simulink model "Quad_Nonlinear_Pitch_Model"  (R2020a)
settings: Solver=ode4  StartTime=0.0  StopTime=5  FixedStep=0.01  RelTol=1e-3
InitFcn:
  | LQIR_Solver;
undefined symbols (not defined in the file or in its folder): B1, B5, Ba, K
settings Model: Creator=Ali  LastModifiedBy=Ali

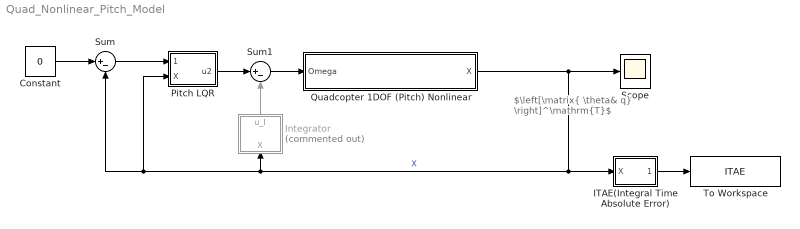
== system Quad_Nonlinear_Pitch_Model ==
  note: $\left[\matrix{ \theta& q} \right]^\mathrm{T}$
  Constant : Constant  Value=0
  ITAE(Integral Time Absolute Error) : Subsystem
  Integrator : Subsystem  Commented=on
  Pitch LQR : Subsystem
  Quadcopter 1DOF (Pitch) Nonlinear : Subsystem  TreatAsAtomicUnit=on
      mask Display: image('Seesaw.png'); % Use "Edit Image" on toolstrip to change.
  Scope : Scope
  Sum : Sum  Inputs=|+-
  Sum1 : Sum  Inputs=|+-
  To Workspace : ToWorkspace  VariableName=ITAE  SaveFormat=Timeseries  SampleTime=-1
  wires:
  Quadcopter 1DOF (Pitch) Nonlinear/1(X) -> Scope/1, Pitch LQR/2(X), Sum/2, Integrator/1(X), ITAE(Integral Time Absolute Error)/1(X)  "X"
  Constant/1 -> Sum/1
  Pitch LQR/1(u2) -> Sum1/1
  Sum1/1 -> Quadcopter 1DOF (Pitch) Nonlinear/1(Omega)
  Integrator/1(u_I) -> Sum1/2
  Sum/1 -> Pitch LQR/1(Error)
  ITAE(Integral Time Absolute Error)/1(ITAE) -> To Workspace/1

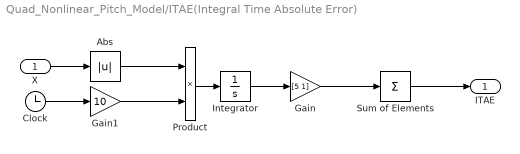
== system Quad_Nonlinear_Pitch_Model/ITAE(Integral Time Absolute Error) ==
  X : Inport
  Abs : Abs
  Clock : Clock
  Gain : Gain  Gain=[5 1]
  Gain1 : Gain  Gain=10
  Integrator : Integrator
  Product : Product
  Sum of Elements : Sum  Inputs=+
  ITAE : Outport
  wires:
  Product/1 -> Integrator/1
  Integrator/1 -> Gain/1
  Clock/1 -> Gain1/1
  Sum of Elements/1 -> ITAE/1
  Abs/1 -> Product/1
  X/1 -> Abs/1
  Gain/1 -> Sum of Elements/1
  Gain1/1 -> Product/2

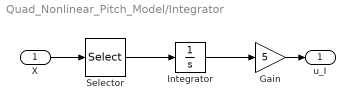
== system Quad_Nonlinear_Pitch_Model/Integrator ==
  X : Inport
  Gain : Gain  Gain=5
  Integrator : Integrator
  Selector : Selector  InputPortWidth=2  IndexOptions=Index vector (dialog)  Indices=[1]  OutputSizes=1
  u_I : Outport
  wires:
  Gain/1 -> u_I/1
  X/1 -> Selector/1
  Integrator/1 -> Gain/1
  Selector/1 -> Integrator/1

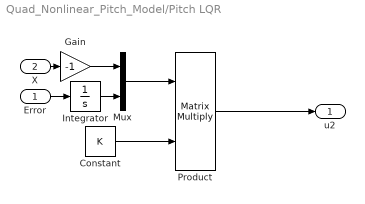
== system Quad_Nonlinear_Pitch_Model/Pitch LQR ==
  Error : Inport
  X : Inport  Port=2
  Constant : Constant  Value=K
  Gain : Gain  Gain=-1
  Integrator : Integrator
  Mux : Mux  Inputs=2
  Product : Product  Multiplication=Matrix(*)
  u2 : Outport
  wires:
  Product/1 -> u2/1
  X/1 -> Gain/1
  Error/1 -> Integrator/1
  Mux/1 -> Product/1
  Constant/1 -> Product/2
  Integrator/1 -> Mux/2
  Gain/1 -> Mux/1

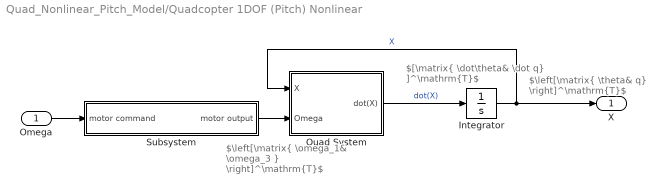
== system Quad_Nonlinear_Pitch_Model/Quadcopter 1DOF (Pitch) Nonlinear ==
  note: $\left[\matrix{ \omega_1& \omega_3 } \right]^\mathrm{T}$
  note: $\left[\matrix{ \theta& q} \right]^\mathrm{T}$
  note: $[\matrix{ \dot\theta& \dot q} ]^\mathrm{T}$
  Omega : Inport
  Integrator : Integrator  InitialCondition=[0.9628, 0]
  Quad System : Subsystem
  Subsystem : Subsystem
  X : Outport
  wires:
  Integrator/1 -> X/1, Quad System/1(X)  "X"
  Quad System/1(dot(X)) -> Integrator/1  "dot(X)"
  Omega/1 -> Subsystem/1(motor command)
  Subsystem/1(motor output) -> Quad System/2(Omega)

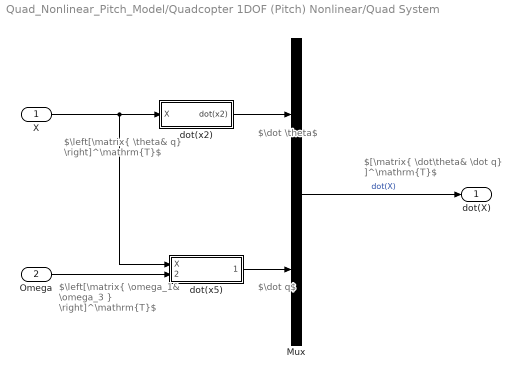
== system Quad_Nonlinear_Pitch_Model/Quadcopter 1DOF (Pitch) Nonlinear/Quad System ==
  note: $\dot \theta$
  note: $\left[\matrix{ \theta& q} \right]^\mathrm{T}$
  note: $[\matrix{ \dot\theta& \dot q} ]^\mathrm{T}$
  note: $\left[\matrix{ \omega_1& \omega_3 } \right]^\mathrm{T}$
  note: $\dot q$
  X : Inport
  Omega : Inport  Port=2
  Mux : Mux  Inputs=2
  dot(x2) : Subsystem
  dot(x5) : Subsystem
  dot(X) : Outport
  wires:
  Mux/1 -> dot(X)/1  "dot(X)"
  dot(x2)/1(dot(x2)) -> Mux/1
  dot(x5)/1(dot(x5)) -> Mux/2
  X/1 -> dot(x5)/1(X), dot(x2)/1(X)
  Omega/1 -> dot(x5)/2(Omega)

== system Quad_Nonlinear_Pitch_Model/Quadcopter 1DOF (Pitch) Nonlinear/Subsystem ==
  motor command : Inport
  Transfer Fcn : TransferFcn  Denominator=[0.15 1]
  motor output : Outport
  wires:
  Transfer Fcn/1 -> motor output/1
  motor command/1 -> Transfer Fcn/1

== system Quad_Nonlinear_Pitch_Model/Quadcopter 1DOF (Pitch) Nonlinear/Quad System/dot(x2) ==
  X : Inport
  1 : Subsystem
  dot(x2) : Outport
  wires:
  X/1 -> 1/1(X)  "X"
  1/1(x5cos(x1)) -> dot(x2)/1

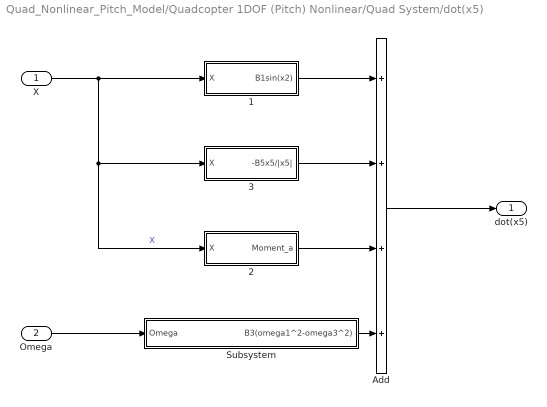
== system Quad_Nonlinear_Pitch_Model/Quadcopter 1DOF (Pitch) Nonlinear/Quad System/dot(x5) ==
  X : Inport
  Omega : Inport  Port=2
  1 : Subsystem
  2 : Subsystem
  3 : Subsystem
  Add : Sum  Inputs=++++
  Subsystem : Subsystem
  dot(x5) : Outport
  wires:
  X/1 -> 2/1(X), 3/1(X), 1/1(X)  "X"
  Omega/1 -> Subsystem/1(Omega)
  Add/1 -> dot(x5)/1
  3/1("-B5x5/|x5| ") -> Add/2
  1/1(B1sin(x2)) -> Add/1
  Subsystem/1(B3(omega1^2-omega3^2)) -> Add/4
  2/1(Moment_a) -> Add/3

== system Quad_Nonlinear_Pitch_Model/Quadcopter 1DOF (Pitch) Nonlinear/Quad System/dot(x2)/1 ==
  X : Inport
  Selector : Selector  InputPortWidth=2  IndexOptions=Index vector (dialog)  Indices=[2]  OutputSizes=1
  x5cos(x1) : Outport
  wires:
  X/1 -> Selector/1  "x"
  Selector/1 -> x5cos(x1)/1

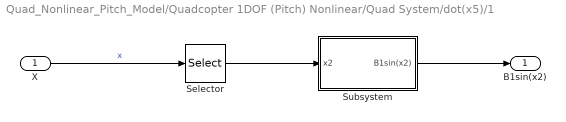
== system Quad_Nonlinear_Pitch_Model/Quadcopter 1DOF (Pitch) Nonlinear/Quad System/dot(x5)/1 ==
  X : Inport
  Selector : Selector  InputPortWidth=2  IndexOptions=Index vector (dialog)  Indices=[1]  OutputSizes=1
  Subsystem : Subsystem
  B1sin(x2) : Outport
  wires:
  X/1 -> Selector/1  "x"
  Subsystem/1(B1sin(x2)) -> B1sin(x2)/1
  Selector/1 -> Subsystem/1(x2)

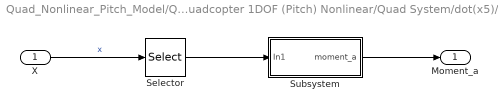
== system Quad_Nonlinear_Pitch_Model/Quadcopter 1DOF (Pitch) Nonlinear/Quad System/dot(x5)/2 ==
  X : Inport
  Selector : Selector  InputPortWidth=2  IndexOptions=Index vector (dialog)  Indices=[1]  OutputSizes=1
  Subsystem : Subsystem
  Moment_a : Outport
  wires:
  X/1 -> Selector/1  "x"
  Subsystem/1(moment_a) -> Moment_a/1
  Selector/1 -> Subsystem/1(In1)

== system Quad_Nonlinear_Pitch_Model/Quadcopter 1DOF (Pitch) Nonlinear/Quad System/dot(x5)/3 ==
  X : Inport
  Selector : Selector  InputPortWidth=2  IndexOptions=Index vector (dialog)  Indices=[2]  OutputSizes=1
  Subsystem : Subsystem
  "-B5x5/|x5| " : Outport
  wires:
  X/1 -> Selector/1  "x"
  Subsystem/1("-B5x5/|x5| ") -> "-B5x5/|x5| "/1
  Selector/1 -> Subsystem/1(x5)

== system Quad_Nonlinear_Pitch_Model/Quadcopter 1DOF (Pitch) Nonlinear/Quad System/dot(x5)/Subsystem ==
  Omega : Inport
  B3(omega1^2-omega3^2) : Outport
  wires:
  Omega/1 -> B3(omega1^2-omega3^2)/1

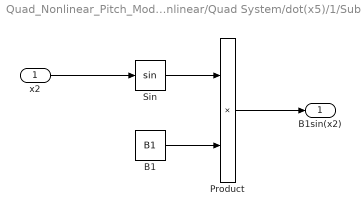
== system Quad_Nonlinear_Pitch_Model/Quadcopter 1DOF (Pitch) Nonlinear/Quad System/dot(x5)/1/Subsystem ==
  x2 : Inport
  B1 : Constant  Value=B1
  Product : Product
  Sin : Trigonometry
  B1sin(x2) : Outport
  wires:
  Product/1 -> B1sin(x2)/1
  x2/1 -> Sin/1
  B1/1 -> Product/2
  Sin/1 -> Product/1

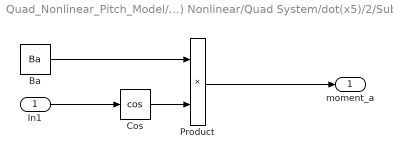
== system Quad_Nonlinear_Pitch_Model/Quadcopter 1DOF (Pitch) Nonlinear/Quad System/dot(x5)/2/Subsystem ==
  In1 : Inport
  Ba : Constant  Value=Ba
  Cos : Trigonometry  Operator=cos
  Product : Product
  moment_a : Outport
  wires:
  Product/1 -> moment_a/1
  Ba/1 -> Product/1
  In1/1 -> Cos/1
  Cos/1 -> Product/2

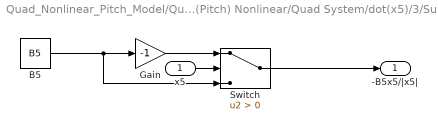
== system Quad_Nonlinear_Pitch_Model/Quadcopter 1DOF (Pitch) Nonlinear/Quad System/dot(x5)/3/Subsystem ==
  x5 : Inport
  B5 : Constant  Value=B5
  Gain : Gain  Gain=-1
  Switch : Switch  Criteria=u2 > Threshold
  "-B5x5/|x5| " : Outport
  wires:
  Switch/1 -> "-B5x5/|x5| "/1
  B5/1 -> Switch/3, Gain/1
  x5/1 -> Switch/2
  Gain/1 -> Switch/1
